simulink subsystem "PieroControlado"  (R2023b)
settings: Solver=VariableStepAuto  StartTime=0.0  StopTime=10.0  RelTol=1e-3
settings Model: Creator=Usuario  LastModifiedBy=Usuario

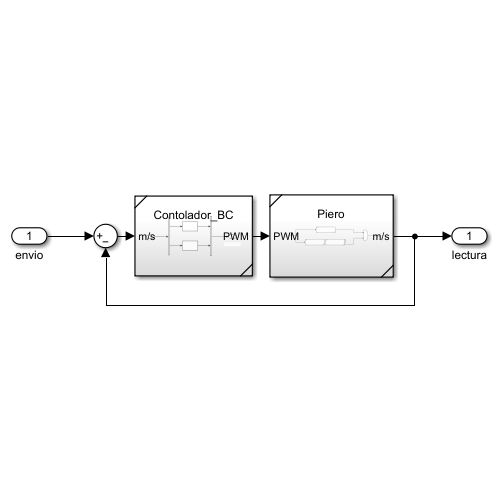
[thumbnail: Simulink's stored preview of the top-level diagram]
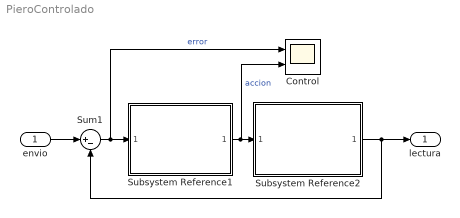
== system PieroControlado ==
  envio : Inport
  Control : Scope  NumInputPorts=2
  Subsystem Reference1 : Subsystem  ReferencedSubsystem=Contolador_BC
  Subsystem Reference2 : Subsystem  ReferencedSubsystem=Piero
  Sum1 : Sum  Inputs=|+-
  lectura : Outport
  wires:
  Subsystem Reference1/1 -> Subsystem Reference2/1, Control/2  "accion"
  Sum1/1 -> Subsystem Reference1/1, Control/1  "error"
  envio/1 -> Sum1/1
  Subsystem Reference2/1 -> lectura/1, Sum1/2
